simulink model "gm_motor_controller"  (R2017a)
settings: Solver=FixedStepDiscrete  StartTime=0.0  StopTime=10.0  RelTol=1e-3
undefined symbols (not defined in the file or in its folder): PWMFreq
settings Model: Creator=mini  LastModifiedBy=mini
settings DataIOCC: SaveOutput=off  SaveTime=off
settings OptimizationCC: BlockReduction=off  ConditionallyExecuteInputs=off  DefaultParameterBehavior=Inlined
settings DebuggingCC: AlgebraicLoopMsg=error  InheritedTsInSrcMsg=none  SingleTaskRateTransMsg=error
settings HardwareCC: ProdBitPerPointer=32  ProdBitPerSizeT=32  ProdBitPerPtrDiffT=32  ProdLargestAtomicFloat=None  ProdIntDivRoundTo=Undefined  ProdEndianess=Unspecified  ProdWordSize=32  ProdHWDeviceType=ASIC/FPGA->ASIC/FPGA  ProdEqTarget=off

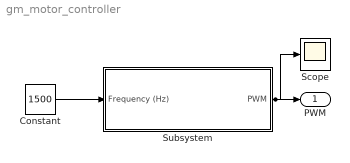
== system gm_motor_controller ==
  Constant : Constant  Value=1500  OutDataTypeStr=uint32
  Scope : Scope
  Subsystem : Subsystem
  PWM : Outport
  wires:
  Constant/1 -> Subsystem/1(Frequency (Hz))
  Subsystem/1(PWM) -> Scope/1, PWM/1

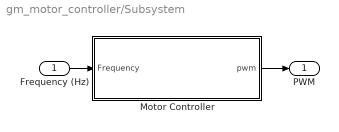
== system gm_motor_controller/Subsystem ==
  Frequency (Hz) : Inport  OutDataTypeStr=uint32
  Motor Controller : Subsystem  mask{fpgaClk=hex2num('4187d78400000000')}
      mask prompts: fpgaClk "FPGA System Clock Freq"
  PWM : Outport
  wires:
  Frequency (Hz)/1 -> Motor Controller/1(Frequency)
  Motor Controller/1(pwm) -> PWM/1

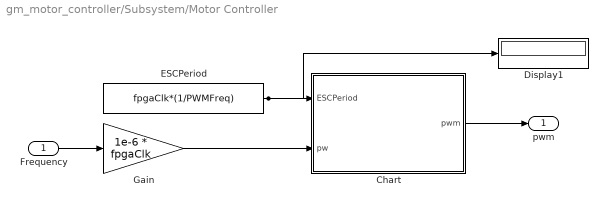
== system gm_motor_controller/Subsystem/Motor Controller ==
  Frequency : Inport
  Chart : Subsystem
  Display1 : Display
  ESCPeriod : Constant  Value=fpgaClk*(1/PWMFreq)  OutDataTypeStr=uint32
  Gain : Gain  Gain=1e-6 * fpgaClk  OutDataTypeStr=Inherit: Same as input
  pwm : Outport
  wires:
  Frequency/1 -> Gain/1
  Chart/1(pwm) -> pwm/1
  ESCPeriod/1 -> Display1/1, Chart/1(ESCPeriod)
  Gain/1 -> Chart/2(pw)

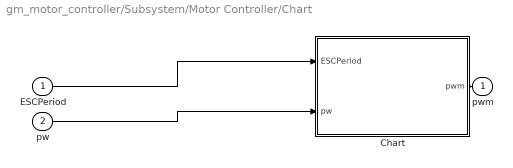
== system gm_motor_controller/Subsystem/Motor Controller/Chart ==
  ESCPeriod : Inport
  pw : Inport  Port=2
  Chart : Stateflow chart  TreatAsAtomicUnit=on
  pwm : Outport
  wires:
  ESCPeriod/1 -> Chart/1(ESCPeriod)
  pw/1 -> Chart/2(pw)
  Chart/1(pwm) -> pwm/1

== stateflow chart gm_motor_controller/Subsystem/Motor Controller/Chart/Chart ==
  settings: executeAtInitialization=1
  state on
    entry: cnt = uint32(0);
    pwm = true;
    during: cnt = cnt + 1;
  state off
    entry: pwm = false;
    during: cnt = cnt + 1;
  (default) -> on
  on -> off : [cnt > pw]
  off -> on : [cnt >= ESCPeriod]
  data: ESCPeriod input uint32; pw input uint32; pwm output boolean; cnt local uint32
